simulink model "Cruise_Model_V13"  (R2024a)
settings: Solver=ode23t  StartTime=0.0  StopTime=2000  RelTol=1e-6
values from neighbouring files (symbols this model uses):
  coefficients =     [alexisignoringme3.mat]    (also in alexisignoringme4.mat)
  K = [-3.60668197653e-15 -4.8519082962e-07 3.58300531153e-06 -0.0035102270316 8.3861852137e-07 3.06276240474 1.22104661107e-16 -0.00351023001393 8.38621571888e-07 3.0627647777 2.01711556188e-16 0.00352147083436 ... (11970 elements, 19x9x70)]    [alexisignoringme2.mat]    (also in alexisignoringme3.mat = [-2.3054870934e-16 -3.29424508508e-08 -2.01640092228e-07 -0.; alexisignoringme4.mat = [-2.3054870934e-16 -3.29424508508e-08 -2.01640092228e-07 -0.; plotLQI_LQR_Comparison.m = Kf(:,:,idx(i)); selectQRfull.m = createGainMat(sysMat, 'QRValsLQR', 'trimUAM1'))
  missionruntime =     [alexisignoringme2.mat]    (also in alexisignoringme3.mat; alexisignoringme4.mat; selectQRfull.m = rmfield(missionruntime, 'rotorTilt'))
  referenceGeo =     [alexisignoringme2.mat]    (also in alexisignoringme3.mat; alexisignoringme4.mat)
  tl = linspace(0, mission.secTime(end), 10000)    [selectQRfull.m]
  U = [2.18842852529e-05 -1.75359463768e-06 7.65324951435e-07 376.143045818 0 0 0 376.144413812 0 0 0 376.143045818 ... (1330 elements, 19x70)]    [alexisignoringme2.mat]    (also in alexisignoringme3.mat = [-1.76080437445e-06 1.51055858734e-07 -7.54037213995e-08 346; createPlots.m = trim.U; selectQRfull.m = reshape(trim.U,size(trim.U,1),[]); trimCost.m = [Z(7:9)' Z(10) 0 rpitch 0              Z(11) 0 rpitch 0     )
  Ut = [0 0 -4.89661324026e-08 0 0 -1504.57476188 -0.000428335964898 -1.57410795509e-09 3.42121377805e-06 0 0 0 ... (450 elements, 9x50)]    [alexisignoringme4.mat]    (also in selectQRfull.m = [U(1:3,:); reshape(trim.Ut, size(trim.Ut,1),[])])
  uvec = [0.1 3.42222222222 6.74444444444 10.0666666667 13.3888888889 16.7111111111 20.0333333333 23.3555555556 26.6777777778 30]    [alexisignoringme2.mat]    (also in alexisignoringme3.mat; alexisignoringme4.mat; selectQRfull.m = zeros(9,10000))
  X = [0.00351655091712 0 -9.99999601592 0 0 0 -4.86374081337e-08 -4.19859407075e-06 -3.62256781384e-09 0.00728108667364 0 -9.23082547646 ... (630 elements, 9x70)]    [alexisignoringme2.mat]    (also in alexisignoringme3.mat = [0.00351658839646 0 -9.99999599468 0 0 0 2.7327442949e-09 -4; alexisignoringme4.mat = [20 0 0 0 0 0 0 0 0]; createPlots.m = trim.X; selectQRfull.m = reshape(trim.X,size(trim.X,1),[]))
  Xes = [24.97004028 0 -1.16861086303 0 0 0 -5.01724449102e-07 -0.0450956248882 0.321650295301]    [alexisignoringme2.mat]    (also in alexisignoringme3.mat = [0.00351658839646 0 -9.99999599468 0 0 0 2.7327442949e-09 -4; alexisignoringme4.mat = [0 0 -1.11199998303 0 0 0 -1.38069247376e-09 1.48137256273e-; plotLQI_LQR_Comparison.m = X(:,idx(i)); selectQRfull.m = X(:,1))
  xvec = zeros(9,10000)    [selectQRfull.m]
undefined symbols (not defined in the file or in its folder): F, Klat, Klong, Light, MIL
libraries: slpidlib x14, aerolibwind2 x8, aerolibatmos2 x4, shared6dof x1
(part 3 of 3)

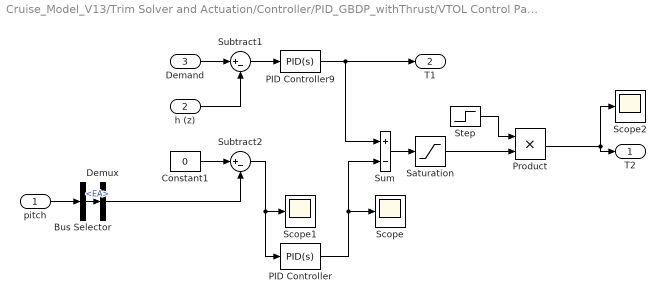
== system Cruise_Model_V13/Trim Solver and Actuation/Controller/PID_GBDP_withThrust/VTOL Control Path ==
  pitch : Inport
  h (z) : Inport  Port=2
  Demand : Inport  Port=3
  Bus Selector : BusSelector  OutputSignals=EA
  Constant1 : Constant  Value=0
  Demux : Demux  Outputs=3
  PID Controller : slpidlib/PID Controller  Controller=PID  Form=Parallel  TimeDomain=Continuous-time  UseExternalTs=off  SampleTime=-1  IntegratorMethod=Forward Euler  FilterMethod=Forward Euler  ControllerParametersSource=internal  P=2347  I=2604  UseKiTs=off  D=519  N=129  UseFilter=on  TunerSelectOption=Transfer Function Based (PID Tuner App)  InitialConditionSource=internal  InitialConditionForIntegrator=0  InitialConditionForFilter=0  DifferentiatorICPrevScaledInput=0  ExternalReset=none  TrackingMode=off  Kt=1  LimitOutput=on  SatLimitsSource=internal  UpperSaturationLimit=800  LowerSaturationLimit=-800  LinearizeAsGain=on  AntiWindupMode=clamping  Kb=1  LimitIntegrator=off  UpperIntegratorSaturationLimit=inf  LowerIntegratorSaturationLimit=-inf  POutMin=[]  POutMax=[]  IOutMin=[]  IOutMax=[]  DOutMin=[]  DOutMax=[]  NOutMin=[]  NOutMax=[]  SumOutMin=[]  SumOutMax=[]  SaturationOutMin=[]  SaturationOutMax=[]  PParamMin=[]  PParamMax=[]  IParamMin=[]  IParamMax=[]  DParamMin=[]  DParamMax=[]  NParamMin=[]  NParamMax=[]  KbParamMin=[]  KbParamMax=[]  KtParamMin=[]  KtParamMax=[]  KbOutMin=[]  KbOutMax=[]  KtOutMin=[]  KtOutMax=[]  IntegratorOutMin=[]  IntegratorOutMax=[]  FilterOutMin=[]  FilterOutMax=[]  SumI1OutMin=[]  SumI1OutMax=[]  SumI2OutMin=[]  SumI2OutMax=[]  SumI3OutMin=[]  SumI3OutMax=[]  SumI4OutMin=[]  SumI4OutMax=[]  SumDOutMin=[]  SumDOutMax=[]  DifferentiatorOutMin=[]  DifferentiatorOutMax=[]  FilterDiffOutCoefMin=[]  FilterDiffOutCoefMax=[]  ReciprocalOutMin=[]  ReciprocalOutMax=[]  SumDenOutMin=[]  SumDenOutMax=[]  SumNumOutMin=[]  SumNumOutMax=[]  DivideOutMin=[]  DivideOutMax=[]  UdiffTsProdOutMin=[]  UdiffTsProdOutMax=[]  NTsProdOutMin=[]  NTsProdOutMax=[]  UintegralTsProdOutMin=[]  UintegralTsProdOutMax=[]  UngainTsProdOutMin=[]  UngainTsProdOutMax=[]  ClampingZeroOutDataTypeStr=Inherit: Inherit via back propagation  ClampingZeroOutMin=[]  ClampingZeroOutMax=[]  FilterDenConstantOutDataTypeStr=Inherit: Inherit via back propagation  FilterDenConstantOutMin=[]  FilterDenConstantOutMax=[]  PCopyOutDataTypeStr=Inherit: Inherit via back propagation  PCopyOutMin=[]  PCopyOutMax=[]  NCopyOutDataTypeStr=Inherit: Inherit via back propagation  NCopyOutMin=[]  NCopyOutMax=[]  IntegratorContinuousStateAttributes=''  IntegratorStateMustResolveToSignalObject=off  IntegratorRTWStateStorageClass=Auto  FilterContinuousStateAttributes=''  FilterStateMustResolveToSignalObject=off  FilterRTWStateStorageClass=Auto  ParallelPVariant=InternalParameters  IdealPVariant=Disabled  IVariant=InternalParameters  DVariant=InternalParameters  IntegratorVariant=Continuous  SatVariant=Enabled  AWVariant=ContClampingParallel  PCopyVariant=Disabled  TRVariant=Disabled  FdbkBlocksVariant=Forward  IdealPFdbkVariant=Disabled  SatFdbkVariant=Disabled  DerivativeFilterVariant=ContFilter  NVariant=InternalParameters  NCopyVariant=Disabled  FilterICVariant=InternalICsFilter  IntegratorICVariant=InternalICs  ExternalResetVariant=Disabled  TRSumVariant=Passthrough  SumFdbkVariant=Disabled  SumVariant=Sum_PID  TsampFilterVariant=InternalTs  TsampNgainVariant=Passthrough  TsampIntegralVariant=Passthrough  ExternalSaturationOutDataTypeStr=Inherit: Same as second input
  PID Controller9 : slpidlib/PID Controller  Controller=PID  Form=Parallel  TimeDomain=Continuous-time  UseExternalTs=off  SampleTime=-1  IntegratorMethod=Forward Euler  FilterMethod=Forward Euler  ControllerParametersSource=internal  P=-174.901958260333  I=-41.0371926298995  UseKiTs=off  D=-183.043785953636  N=27.3346026399604  UseFilter=on  TunerSelectOption=Transfer Function Based (PID Tuner App)  InitialConditionSource=internal  InitialConditionForIntegrator=0  InitialConditionForFilter=0  DifferentiatorICPrevScaledInput=0  ExternalReset=none  TrackingMode=off  Kt=1  LimitOutput=on  SatLimitsSource=internal  UpperSaturationLimit=2000  LowerSaturationLimit=0  LinearizeAsGain=off  AntiWindupMode=clamping  Kb=1  LimitIntegrator=off  UpperIntegratorSaturationLimit=inf  LowerIntegratorSaturationLimit=-inf  POutMin=[]  POutMax=[]  IOutMin=[]  IOutMax=[]  DOutMin=[]  DOutMax=[]  NOutMin=[]  NOutMax=[]  SumOutMin=[]  SumOutMax=[]  SaturationOutMin=[]  SaturationOutMax=[]  PParamMin=[]  PParamMax=[]  IParamMin=[]  IParamMax=[]  DParamMin=[]  DParamMax=[]  NParamMin=[]  NParamMax=[]  KbParamMin=[]  KbParamMax=[]  KtParamMin=[]  KtParamMax=[]  KbOutMin=[]  KbOutMax=[]  KtOutMin=[]  KtOutMax=[]  IntegratorOutMin=[]  IntegratorOutMax=[]  FilterOutMin=[]  FilterOutMax=[]  SumI1OutMin=[]  SumI1OutMax=[]  SumI2OutMin=[]  SumI2OutMax=[]  SumI3OutMin=[]  SumI3OutMax=[]  SumI4OutMin=[]  SumI4OutMax=[]  SumDOutMin=[]  SumDOutMax=[]  DifferentiatorOutMin=[]  DifferentiatorOutMax=[]  FilterDiffOutCoefMin=[]  FilterDiffOutCoefMax=[]  ReciprocalOutMin=[]  ReciprocalOutMax=[]  SumDenOutMin=[]  SumDenOutMax=[]  SumNumOutMin=[]  SumNumOutMax=[]  DivideOutMin=[]  DivideOutMax=[]  UdiffTsProdOutMin=[]  UdiffTsProdOutMax=[]  NTsProdOutMin=[]  NTsProdOutMax=[]  UintegralTsProdOutMin=[]  UintegralTsProdOutMax=[]  UngainTsProdOutMin=[]  UngainTsProdOutMax=[]  ClampingZeroOutDataTypeStr=Inherit: Inherit via back propagation  ClampingZeroOutMin=[]  ClampingZeroOutMax=[]  FilterDenConstantOutDataTypeStr=Inherit: Inherit via back propagation  FilterDenConstantOutMin=[]  FilterDenConstantOutMax=[]  PCopyOutDataTypeStr=Inherit: Inherit via back propagation  PCopyOutMin=[]  PCopyOutMax=[]  NCopyOutDataTypeStr=Inherit: Inherit via back propagation  NCopyOutMin=[]  NCopyOutMax=[]  IntegratorContinuousStateAttributes=''  IntegratorStateMustResolveToSignalObject=off  IntegratorRTWStateStorageClass=Auto  FilterContinuousStateAttributes=''  FilterStateMustResolveToSignalObject=off  FilterRTWStateStorageClass=Auto  ParallelPVariant=InternalParameters  IdealPVariant=Disabled  IVariant=InternalParameters  DVariant=InternalParameters  IntegratorVariant=Continuous  SatVariant=Enabled  AWVariant=ContClampingParallel  PCopyVariant=Disabled  TRVariant=Disabled  FdbkBlocksVariant=Forward  IdealPFdbkVariant=Disabled  SatFdbkVariant=Disabled  DerivativeFilterVariant=ContFilter  NVariant=InternalParameters  NCopyVariant=Disabled  FilterICVariant=InternalICsFilter  IntegratorICVariant=InternalICs  ExternalResetVariant=Disabled  TRSumVariant=Passthrough  SumFdbkVariant=Disabled  SumVariant=Sum_PID  TsampFilterVariant=InternalTs  TsampNgainVariant=Passthrough  TsampIntegralVariant=Passthrough  ExternalSaturationOutDataTypeStr=Inherit: Same as second input
  Product : Product
  Saturation : Saturate  UpperLimit=9000  LowerLimit=0
  Scope : Scope
  Scope1 : Scope
  Scope2 : Scope
  Step : Step  Time=max(mission.trans.t)  Before=1  After=0  SampleTime=0
  Subtract1 : Sum  Inputs=|+-
  Subtract2 : Sum  Inputs=|+-
  Sum : Sum  Inputs=+-
  T2 : Outport
  T1 : Outport  Port=2
  wires:
  Demand/1 -> Subtract1/1
  h (z)/1 -> Subtract1/2
  Subtract1/1 -> PID Controller9/1
  Constant1/1 -> Subtract2/1
  pitch/1 -> Bus Selector/1
  Subtract2/1 -> PID Controller/1, Scope1/1
  PID Controller9/1 -> Sum/1, T1/1
  Sum/1 -> Saturation/1
  PID Controller/1 -> Sum/2, Scope/1
  Bus Selector/1 -> Demux/1  "<EA>"
  Demux/2 -> Subtract2/2
  Product/1 -> T2/1, Scope2/1
  Saturation/1 -> Product/2
  Step/1 -> Product/1

== system Cruise_Model_V13/Trim Solver and Actuation/Controller/Trim Solver/Saturation2 ==
  In1 : Inport
  Demux3 : Demux  Outputs=9
  Mux : Mux  Inputs=9
  Saturation : Saturate
  Saturation1 : Saturate
  Saturation2 : Saturate
  Saturation3 : Saturate  UpperLimit=1.6*150*9.81
  Saturation4 : Saturate  UpperLimit=1.6*150*9.81
  Saturation5 : Saturate  UpperLimit=1.6*150*9.81
  Saturation6 : Saturate  UpperLimit=700
  Saturation7 : Saturate  UpperLimit=700
  Saturation8 : Saturate  UpperLimit=700
  U : Outport
  wires:
  In1/1 -> Demux3/1
  Mux/1 -> U/1
  Demux3/1 -> Saturation/1
  Saturation/1 -> Mux/1
  Saturation1/1 -> Mux/2
  Demux3/2 -> Saturation1/1
  Saturation2/1 -> Mux/3
  Demux3/3 -> Saturation2/1
  Demux3/4 -> Saturation3/1
  Saturation3/1 -> Mux/4
  Demux3/5 -> Saturation4/1
  Saturation4/1 -> Mux/5
  Saturation5/1 -> Mux/6
  Demux3/6 -> Saturation5/1
  Saturation6/1 -> Mux/7
  Demux3/7 -> Saturation6/1
  Saturation7/1 -> Mux/8
  Demux3/8 -> Saturation7/1
  Saturation8/1 -> Mux/9
  Demux3/9 -> Saturation8/1

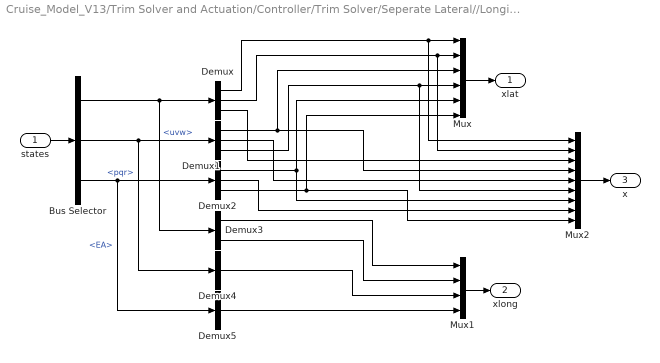
== system Cruise_Model_V13/Trim Solver and Actuation/Controller/Trim Solver/Seperate Lateral//Longitudinal ==
  states : Inport
  Bus Selector : BusSelector  OutputSignals=uvw,pqr,EA
  Demux{,1..5} (6 alike) : Demux  Outputs=3
  Mux : Mux  Inputs=6
  Mux1 : Mux
  Mux2 : Mux  Inputs=9
  xlat : Outport
  xlong : Outport  Port=2
  x : Outport  Port=3
  wires:
  states/1 -> Bus Selector/1
  Mux/1 -> xlat/1
  Mux1/1 -> xlong/1
  Bus Selector/1 -> Demux/1, Demux3/1  "<uvw>"
  Bus Selector/2 -> Demux1/1, Demux4/1  "<pqr>"
  Bus Selector/3 -> Demux5/1, Demux2/1  "<EA>"
  Demux/1 -> Mux2/1, Mux/1
  Demux/2 -> Mux2/2, Mux/2
  Demux1/1 -> Mux2/4, Mux/3
  Demux1/3 -> Mux2/6, Mux/4
  Demux2/1 -> Mux2/7, Mux/5
  Demux2/3 -> Mux2/9, Mux/6
  Demux3/1 -> Mux1/1
  Demux3/3 -> Mux1/2
  Demux4/2 -> Mux1/3
  Demux5/2 -> Mux1/4
  Mux2/1 -> x/1
  Demux/3 -> Mux2/3
  Demux1/2 -> Mux2/5
  Demux2/2 -> Mux2/8

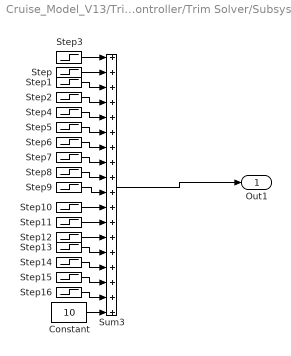
== system Cruise_Model_V13/Trim Solver and Actuation/Controller/Trim Solver/Subsystem ==
  Constant : Constant  Value=10
  Step : Step  Time=60  Before=1  After=2  SampleTime=0
  Step1 : Step  Time=180  SampleTime=0
  Step10 : Step  Time=660  SampleTime=0
  Step11 : Step  Time=720  SampleTime=0
  Step12 : Step  Time=780  SampleTime=0
  Step13 : Step  Time=1000  SampleTime=0
  Step14 : Step  Time=1260  SampleTime=0
  Step15 : Step  Time=1320  SampleTime=0
  Step16 : Step  Time=1400  SampleTime=0
  Step2 : Step  Time=240  SampleTime=0
  Step3 : Step  Time=120  SampleTime=0
  Step4 : Step  Time=300  SampleTime=0
  Step5 : Step  Time=360  SampleTime=0
  Step6 : Step  Time=420  SampleTime=0
  Step7 : Step  Time=480  SampleTime=0
  Step8 : Step  Time=540  SampleTime=0
  Step9 : Step  Time=600  SampleTime=0
  Sum3 : Sum  Inputs=++++++++++++++++++
  Out1 : Outport
  wires:
  Step/1 -> Sum3/2
  Step2/1 -> Sum3/4
  Step3/1 -> Sum3/1
  Step5/1 -> Sum3/6
  Step8/1 -> Sum3/9
  Step1/1 -> Sum3/3
  Sum3/1 -> Out1/1
  Step6/1 -> Sum3/7
  Step4/1 -> Sum3/5
  Step7/1 -> Sum3/8
  Step9/1 -> Sum3/10
  Step10/1 -> Sum3/11
  Step11/1 -> Sum3/12
  Step12/1 -> Sum3/13
  Step13/1 -> Sum3/14
  Step14/1 -> Sum3/15
  Step15/1 -> Sum3/16
  Step16/1 -> Sum3/17
  Constant/1 -> Sum3/18

== system Cruise_Model_V13/Trim Solver and Actuation/Controller/PID_GBDP_withThrust/Altitude Control Path/Step demand for testing ==
  In1 : Inport
  Mux1 : Mux  Inputs=2
  Scope2 : Scope
  Scope4 : Scope
  Step1 : Step  Time=60  Before=-500  After=-490  SampleTime=0
  Step2 : Step  Time=80  After=-10  SampleTime=0
  Step3 : Step  Time=120  After=20  SampleTime=0
  Step4 : Step  Time=120  After=20  SampleTime=0
  Sum : Sum  Inputs=++++
  To Workspace : ToWorkspace  VariableName=altitudeResponse  SaveFormat=Timeseries  SampleTime=-1
  Out1 : Outport
  wires:
  Step3/1 -> Sum/3
  Mux1/1 -> To Workspace/1, Scope4/1
  Sum/1 -> Out1/1, Mux1/1
  Step4/1 -> Sum/4
  Step1/1 -> Sum/1
  In1/1 -> Mux1/2, Scope2/1
  Step2/1 -> Sum/2

== system Cruise_Model_V13/Trim Solver and Actuation/Controller/PID_GBDP_withThrust/Course Angle Control Path/Step demand for testing2 ==
  Va : Inport
  Mux1 : Mux  Inputs=2
  Scope2 : Scope
  Scope4 : Scope
  Step1 : Step  Time=60  Before=0.1  After=0.2  SampleTime=0
  Step2 : Step  Time=80  After=-0.4  SampleTime=0
  Step3 : Step  Time=120  After=-0.2  SampleTime=0
  Step4 : Step  Time=100  After=0.6  SampleTime=0
  Step5 : Step  Time=140  After=-0.4  SampleTime=0
  Sum : Sum  Inputs=+++++
  To Workspace : ToWorkspace  VariableName=headingAngleResponse  SaveFormat=Timeseries  SampleTime=-1
  Out1 : Outport
  wires:
  Step5/1 -> Sum/5
  Step3/1 -> Sum/3
  Mux1/1 -> To Workspace/1, Scope4/1
  Sum/1 -> Out1/1, Mux1/1
  Step4/1 -> Sum/4
  Step1/1 -> Sum/1
  Va/1 -> Mux1/2, Scope2/1
  Step2/1 -> Sum/2

== system Cruise_Model_V13/Trim Solver and Actuation/Controller/PID_GBDP_withThrust/Subsystem/Step demand for testing1 ==
  Va : Inport
  Mux1 : Mux  Inputs=2
  Scope2 : Scope
  Scope4 : Scope
  Step1 : Step  Time=60  Before=25  After=31  SampleTime=0
  Step2 : Step  Time=80  After=-3  SampleTime=0
  Step3 : Step  Time=120  After=-5  SampleTime=0
  Step4 : Step  Time=100  After=8  SampleTime=0
  Step5 : Step  Time=140  After=-2  SampleTime=0
  Sum : Sum  Inputs=+++++
  To Workspace : ToWorkspace  VariableName=airspeedResponse  SaveFormat=Timeseries  SampleTime=-1
  Out1 : Outport
  wires:
  Step2/1 -> Sum/2
  Va/1 -> Scope2/1, Mux1/2
  Step1/1 -> Sum/1
  Step4/1 -> Sum/4
  Sum/1 -> Mux1/1, Out1/1
  Mux1/1 -> Scope4/1, To Workspace/1
  Step3/1 -> Sum/3
  Step5/1 -> Sum/5

== matlab function Cruise_Model_V13/Trim Solver and Actuation/Controller/Trim Solver/MATLAB Function5 ==
  data: uref_lat output; Ue input; K input; time input; mission parameter; uref_long output; uref output; xerr input; U output
function [uref_lat, uref_long, uref, U] = fcn(Ue, K, time, mission, xerr)

t = linspace(0, mission.secTime(end), size(Ue,1));
[~, idx] = min(abs(t - time));

uref = Ue(:,idx);
uref_lat = uref([1 2 4 6 7 9]);
uref_long = uref([1 3 5 8]);
u = K(:,:,idx)*xerr;

U = uref + u;

== matlab function Cruise_Model_V13/Trim Solver and Actuation/Controller/Trim Solver/MATLAB Function2 ==
  data: Uei output; ulat output; ulong output; U output; Ue input; time input; xlat input; xlong input; mission parameter; Klat input; Klong input
function [Uei, ulat, ulong, U] = fcn(Ue, time, xlat, xlong, mission, Klat, Klong)

t = linspace(0, mission.secTime(end), size(Ue,2));
[~, idx] = min(abs(t - time));

ulat = -Klat(:,:,idx)*xlat;
ulong = -Klong(:,:,idx)*xlong;
u = (ulat + ulong)./2;

U = Ue(:,idx) + u;
Uei = Ue(:,idx);

== matlab function Cruise_Model_V13/Aircraft Dynamics/Aerodynamic Forces and Moments/MATLAB Function ==
  data: Fb output; Mcg output; coeff input Bus: coeff; u input; alpha input; beta input; V input; rho input; X input; refGeo parameter; m parameter; thrust input; cg parameter
function [Fb,Mcg] = aeroDyn(coeff, u, alpha, beta, V, rho, X, refGeo, m, thrust, cg)
% Function aeroDyn simulates ....

%% Setting up intermediate variables
b = refGeo.bref;
S = refGeo.Sref;
c = refGeo.cref;

Q = 0.5*rho*V^2; % Dynamic pressure Q

ndc = c/(2*V);
ndb = b/(2*V);

%% Seperating vectors (BFR)
uvw = X(1:3); % Translational velocity vector
pqr = X(4:6); % Angular velocity vector
EA = X(7:end);

%% Handle Stall

%% Non-dimensional Aerodynamic Force Coefficients
% In wind axis
% Lift
CL = applyDeriv(coeff.CL0, coeff.CLa, coeff.CLb, coeff.CLn, 0, coeff.CLq, 0, u, alpha, beta, pqr, ndc);

% Drag 
CD = applyDeriv(coeff.CD0, coeff.CDa, coeff.CDb, coeff.CDn, 0, 0, 0, u, alpha, beta, pqr, ndc);

% Sideforce
CY = applyDeriv(0, coeff.CYa, coeff.CYb, coeff.CYn, coeff.CYp, 0, coeff.CYr, u, alpha, beta, pqr, ndb);

if abs(alpha) > 14.5*(pi/180)
    CL = 0;
    CD = coeff.CD0;
    CY = 0;
end

%% Rotate wind to body
Faw = [-max(CD,0); CY; -CL].*Q*S; % Force vector in the stability frame

Rwb = [cos(alpha)*cos(beta), -cos(alpha)*sin(beta), -sin(alpha);  
       sin(beta)           ,  cos(beta)           ,  0         ; 
       cos(beta)*sin(alpha), -sin(alpha)*sin(beta),  cos(alpha)];

Fab = Rwb*Faw; % aerodynamic force on body

%% Aerodynamic Moment about CG
% In Fb, with moments taken about the centre of gravity

% Roll
Cl = applyDeriv(0, coeff.Cla, coeff.Clb, coeff.Cln, coeff.Clp, 0, coeff.Clr, u, alpha, beta, pqr, ndb);

% Pitch
Cm = applyDeriv(coeff.Cm0, coeff.Cma, coeff.Cmb, coeff.Cmn, 0, coeff.Cmq, 0, u, alpha, beta, pqr, ndc);

% Yaw
Cn = applyDeriv(0, coeff.Cna, coeff.Cnb, coeff.Cnn, coeff.Cnp, 0, coeff.Cnr, u, alpha, beta, pqr, ndb);

if abs(alpha) > 20*(pi/180)
    Cm = 0;
    Cn = 0;
    Cl = 0;
end

Ma = [b*Cl; c*Cm; b*Cn].*Q*S;

%% Propulsion Effects
% Moment and forces induced by throttle
FTb = u(4:6);
MTcg = u(7:9);

% Gravity Effects
Fgb = [-9.81*sin(X(8))          ; % Body frame
        9.81*cos(X(8))*sin(X(7));
        9.81*cos(X(8))*cos(X(7))]*m; % ASSUMPTION: Constant Mass

%% Out
Rbe = body2earth(X(7), X(8), X(9));

Fb = FTb + Fgb + Fab;
Mcg = MTcg + Ma;

forces = [FTb; Fgb; Fab; Rbe*Fb];
aero = [CL; CD; Cm];
uvw_e = Rbe*X(1:3);

end

%% Extra functions

function C = applyDeriv(C0, Ca, Cb, Cn, Cp, Cq, Cr, u, alpha, beta, pqr, nd)
% function applyDeriv calculates the coefficient C from the derivatives C0,
% Ca, Cb, Cn wrt 0, alpha, beta and control (n), respectively.

    C_nc = C0 + Ca*alpha + Cb*beta + Cp*pqr(1)*nd + Cq*pqr(2)*nd + Cr*pqr(3)*nd; % lift coefficient no control
    
    C_c = (Cn.*u(1:length(Cn)))';

    C = C_nc + sum(C_c);

end

== matlab function Cruise_Model_V13/Trim Solver and Actuation/Controller/Trim Solver/MATLAB Function1 ==
  data: idx output; Xe input; idx input; mission parameter; xd output; time input; t input; tl input; xvec input; idxl output
function [idx, xd, idxl] = fcn(Xe, idx, mission, time, t, tl, xvec)

[~, idx] = min(abs(t - time));
[~, idxl] = min(abs(tl - time));

xd = xvec(:,idxl);

== matlab function Cruise_Model_V13/Trim Solver and Actuation/Controller/Trim Solver/MATLAB Function3 ==
  data: uref output; Ue input; K input; idx input; k output; uvec input; idxl input
function [uref, k]  = fcn(Ue, K, idx, uvec, idxl)

uref = Ue(:,idx);
uref = uvec(:,idxl);
k = K(:,:,idx);
